simulink model "DifferentialDriveRestricted"  (Simulink 8.7)
settings: Solver=VariableStepAuto  StartTime=0.0  StopTime=10.0  RelTol=1e-3
settings Model: Creator=maximilian  LastModifiedBy=maximilian
settings DataIOCC: LimitDataPoints=off  SaveFormat=Dataset
settings DebuggingCC: UnderspecifiedInitializationDetection=Simplified  MergeDetectMultiDrivingBlocksExec=error
settings HardwareCC: ProdBitPerPointer=64  ProdLargestAtomicFloat=Float  ProdIntDivRoundTo=Zero  ProdEndianess=LittleEndian  ProdWordSize=64  ProdHWDeviceType=Intel->x86-64 (Windows64)
settings ModelReferenceCC: PropagateSignalLabelsOutOfModel=on
settings ConfigComp: CovModelRefEnable=off

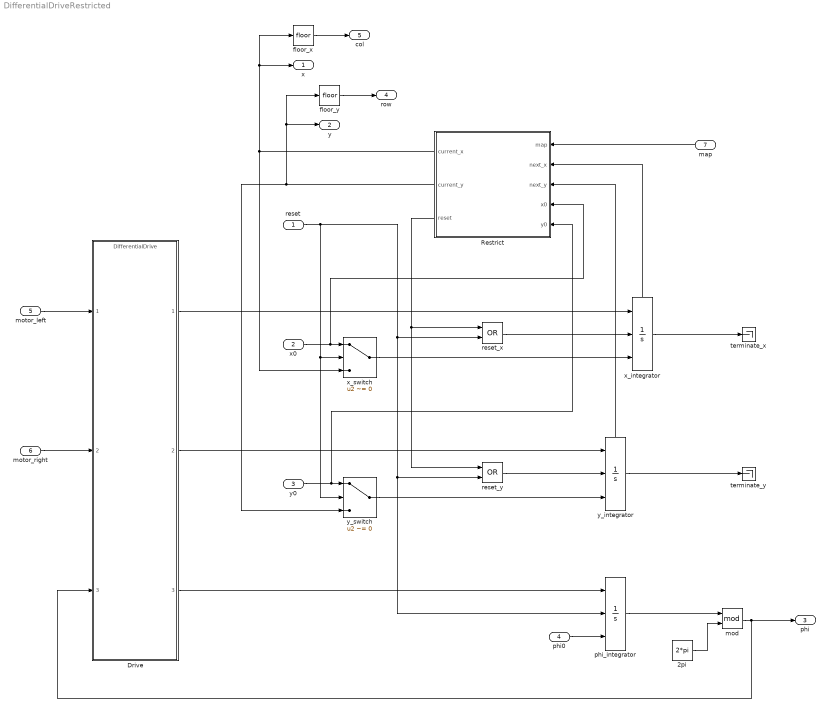
== system DifferentialDriveRestricted ==
  reset : Inport
  x0 : Inport  Port=2
  y0 : Inport  Port=3
  phi0 : Inport  Port=4
  motor_left : Inport  Port=5
  motor_right : Inport  Port=6
  map : Inport  Port=7  PortDimensions=[100 100]
  2pi : Constant  Value=2*pi
  Drive : ModelReference  ModelNameDialog=DifferentialDrive.mdl  SimulationMode=Normal  ModelReferenceVersion=1.13
  Restrict : Stateflow chart  TreatAsAtomicUnit=on
  floor_x : Rounding
  floor_y : Rounding
  mod : Math  Operator=mod  SaturateOnIntegerOverflow=on
  phi_integrator : Integrator  ExternalReset=rising  InitialConditionSource=external
  reset_x : Logic  Operator=OR  AllPortsSameDT=off  OutDataTypeStr=boolean
  reset_y : Logic  Operator=OR  AllPortsSameDT=off  OutDataTypeStr=boolean
  terminate_x : Terminator
  terminate_y : Terminator
  x_integrator : Integrator  ExternalReset=rising  InitialConditionSource=external  ShowStatePort=on
  x_switch : Switch  Criteria=u2 ~= 0
  y_integrator : Integrator  ExternalReset=rising  InitialConditionSource=external  ShowStatePort=on
  y_switch : Switch  Criteria=u2 ~= 0
  "x " : Outport
  y : Outport  Port=2
  "phi " : Outport  Port=3
  row : Outport  Port=4
  col : Outport  Port=5
  wires:
  Drive/1 -> x_integrator/1
  Drive/2 -> y_integrator/1
  Drive/3 -> phi_integrator/1
  phi_integrator/1 -> mod/1
  motor_left/1 -> Drive/1
  motor_right/1 -> Drive/2
  reset_x/1 -> x_integrator/2
  Restrict/3(reset) -> reset_y/1, reset_x/1
  reset_y/1 -> y_integrator/2
  x_switch/1 -> x_integrator/3
  reset/1 -> phi_integrator/2, reset_y/2, reset_x/2, x_switch/2, y_switch/2
  y_switch/1 -> y_integrator/3
  x0/1 -> Restrict/4(x0), x_switch/1
  x_integrator/State -> Restrict/2(next_x)
  y_integrator/State -> Restrict/3(next_y)
  phi0/1 -> phi_integrator/3
  y0/1 -> Restrict/5(y0), y_switch/1
  map/1 -> Restrict/1(map)
  floor_x/1 -> col/1
  Restrict/1(current_x) -> floor_x/1, "x "/1, x_switch/3
  floor_y/1 -> row/1
  Restrict/2(current_y) -> y/1, floor_y/1, y_switch/3
  x_integrator/1 -> terminate_x/1
  y_integrator/1 -> terminate_y/1
  mod/1 -> "phi "/1, Drive/3
  2pi/1 -> mod/2

== stateflow chart Restrict ==
  state Reset
  state Start
  (default) -> Start : {
      | 	current_x = x0; current_y = y0; reset = 0;
      | 	x = current_x; y = current_y;
      | 	col = floor(x) + 1; row = floor(y) + 1
      | }
  Start -> Start [order 2] : {
      | 	x = next_x; y = next_y;
      | 	col = floor(y); row = floor(x) ;
      | 	current_x = x;
      | 	current_y = y;
      | }
  Reset -> Start : {reset = 0;}
  Start -> Reset [order 1] : [map(floor(next_y), floor(next_x)) ~= 0 && floor(next_y) ~= row && floor(next_x) ~= col]{
      | 	reset = 1;
      | 	current_x = x;
      | 	current_y = y;
      | }
  data: map input double size=[100 100]; next_x input double; next_y input double; current_x output double =0; current_y output double =0; reset output double =0; x local double; y local double; x0 input double; y0 input double; col local double; row local double
